simulink model "Ex_3"  (R2020a)
settings: Solver=VariableStepAuto  StartTime=0.0  StopTime=tstop  RelTol=1e-3
values from neighbouring files (symbols this model uses):
  iLo = 0    [m2.m]    (also in m3.m)
  L = 0.1    [m2.m]    (also in m3.m = 0.04)
  R = 0.4    [m3.m]
  Vac = 100    [m3.m]
  we = 314    [m3.m]
settings Model: Creator=abhin  LastModifiedBy=abhin

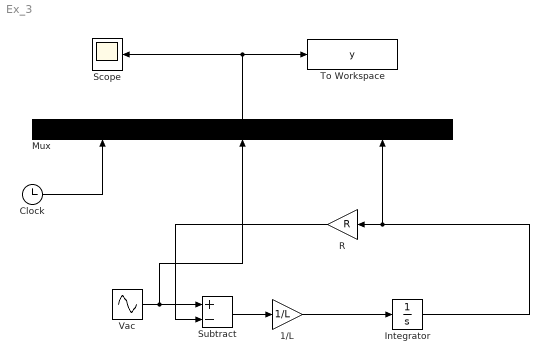
== system Ex_3 ==
  1/L : Gain  Gain=1/L
  Clock : Clock
  Integrator : Integrator  InitialCondition=iLo
  Mux : Mux  Inputs=3
  R : Gain  Gain=R
  Scope : Scope
  Subtract : Sum  Inputs=+-
  To Workspace : ToWorkspace  VariableName=y  SaveFormat=Structure  SampleTime=-1
      settings: Save2DSignal=2-D array (concatenate along first dimension)
  Vac : Sin  Amplitude=Vac  Frequency=we  SampleTime=1e-6
  wires:
  1/L/1 -> Integrator/1
  Subtract/1 -> 1/L/1
  Integrator/1 -> Mux/3, R/1
  R/1 -> Subtract/2
  Mux/1 -> To Workspace/1, Scope/1
  Clock/1 -> Mux/1
  Vac/1 -> Subtract/1, Mux/2
